simulink model "kompl_fft"  (Simulink 4.00)
settings: Solver=ode45  StartTime=0.0  StopTime=100  RelTol=1e-3
values from neighbouring files (symbols this model uses):
  hh = remez(Nfilter, [0.02, 0.48]*2, [1 1], 'Hilbert')    [kompl_fft_p.m]
  Ts = 1/fs    [abtast1.m]    (also in fourier4.m = 0.001; fourier5.m = 0.00125; kompl_fft_p.m = 0.001)
undefined symbols (not defined in the file or in its folder): get
libraries: dsparch3 x1, dspsigops x1, dspsnks3 x1
settings Model: LastModifiedBy=Administrator  BlockReductionOpt=off

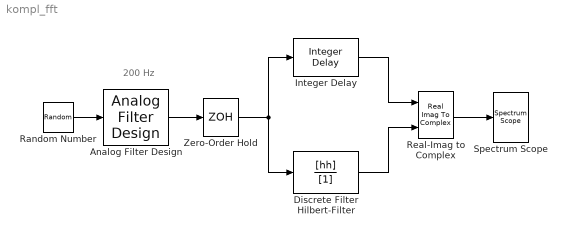
== system kompl_fft ==
  note: 200 Hz
  Analog Filter Design : dsparch3/Analog Filter Design  method=Chebyshev I  filttype=Lowpass  N=8  Wlo=2*pi*200  Whi=80  Rp=1  Rs=40
  Discrete Filter Hilbert-Filter : DiscreteFilter  Numerator=[hh]  Denominator=[1]  SampleTime=Ts  Realization=auto
  Integer Delay : dspsigops/Integer Delay  delay=delay  ic=0
  Random Number : RandomNumber  Mean=0  Variance=1  Seed=0  SampleTime=0
  Real-Imag to Complex : RealImagToComplex  Input=RealAndImag  ConstantPart=0
  Spectrum Scope : dspsnks3/Spectrum Scope  ScopeProperties=off  Domain=Frequency  HorizSpan=1  UseBuffer=on  BufferSize=256  Overlap=32  inpFftLenInherit=off  FFTlength=128  numAvg=32  DisplayProperties=off  AxisGrid=on  Memory=off  FrameNumber=on  AxisLegend=off  AxisZoom=off  OpenScopeAtSimStart=on  OpenScopeImmediately=off  FigPos=get(0,'defaultfigureposition')  AxisProperties=on  XUnits=Hertz  XRange=[0...Fs]  InheritXIncr=off  XIncr=Ts  XLabel=Samples  YUnits=dB  YLabel=Magnitude, dB  LineProperties=off
      link override Optional Buffering/Buffer: N=BufferSize  V=Overlap  ic=0
      settings: YMin=6.85108357021385e-013  YMax=6.30619501031431
  Zero-Order Hold : ZeroOrderHold  SampleTime=Ts
  wires:
  Random Number/1 -> Analog Filter Design/1
  Analog Filter Design/1 -> Zero-Order Hold/1
  Discrete Filter Hilbert-Filter/1 -> Real-Imag to Complex/2
  Integer Delay/1 -> Real-Imag to Complex/1
  Real-Imag to Complex/1 -> Spectrum Scope/1
  Zero-Order Hold/1 -> Integer Delay/1, Discrete Filter Hilbert-Filter/1
